simulink model "coordinate_transform_quat"  (R2018a)
settings: Solver=VariableStepAuto  StartTime=0.0  StopTime=10.0  RelTol=1e-3
settings Model: Creator=lamy  LastModifiedBy=lamy

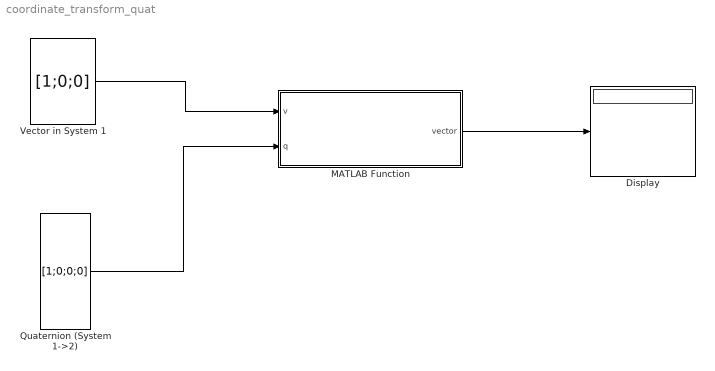
== system coordinate_transform_quat ==
  Display : Display
  MATLAB Function : MATLAB Function  TreatAsAtomicUnit=on
  Quaternion (System 1->2) : Constant  Value=[1;0;0;0]  VectorParams1D=off
  Vector in System 1 : Constant  Value=[1;0;0]  VectorParams1D=off
  wires:
  Quaternion (System 1->2)/1 -> MATLAB Function/2(q)
  Vector in System 1/1 -> MATLAB Function/1(v)
  MATLAB Function/1(vector) -> Display/1

== matlab function coordinate_transform_quat/MATLAB Function ==
  data: v input; vector output; q input
function vector = coordinate_transform_quat(v,q)
qo=q(1);
qvec=q(2:4);
vector = 2*qvec*(dot(qvec,v)) + (qo^2 - dot(qvec,qvec))*v + 2*qo*cross(v,qvec);
